simulink model "Planar_Full_System_NL"  (R2016a)
settings: Solver=ode45  StartTime=0.0  StopTime=2  RelTol=1e-3
values from neighbouring files (symbols this model uses):
  T_x_AP = 0    [Computation.m]
  T_y_AP = 0    [Computation.m]
  T_z_AP = 0    [Computation.m]
  x_AP = [0;0;0;0]    [Computation.m]
undefined symbols (not defined in the file or in its folder): K_xz, K_yz
settings Model: Creator=Florian  LastModifiedBy=Florian

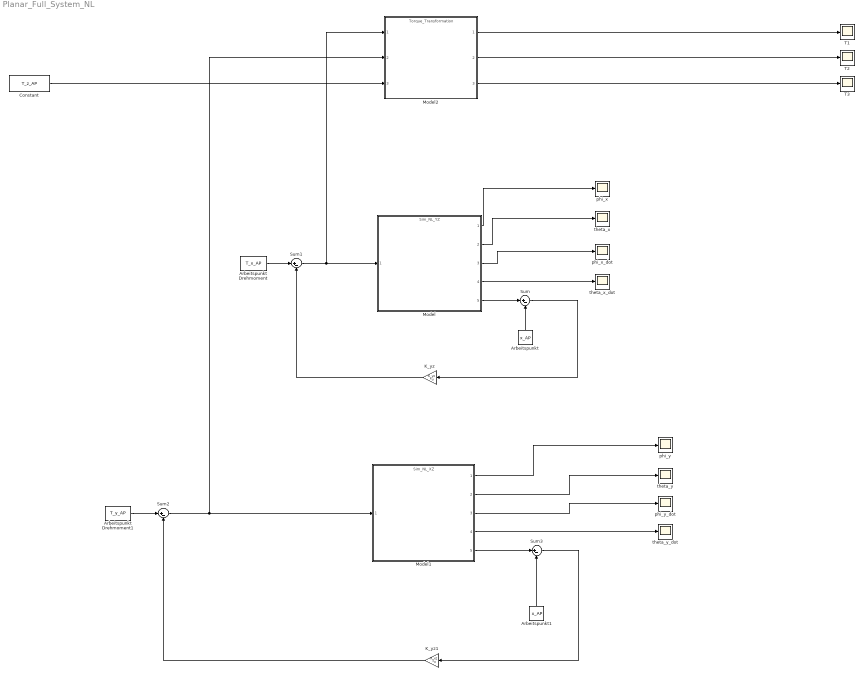
== system Planar_Full_System_NL ==
  Arbeitspunkt : Constant  Value=x_AP
  Arbeitspunkt Drehmoment : Constant  Value=T_x_AP
  Arbeitspunkt Drehmoment1 : Constant  Value=T_y_AP
  Arbeitspunkt1 : Constant  Value=x_AP
  Constant : Constant  Value=T_z_AP
  K_yz : Gain  Gain=K_yz  Multiplication=Matrix(K*u) (u vector)
  K_yz1 : Gain  Gain=K_xz  Multiplication=Matrix(K*u) (u vector)
  Model : ModelReference  ModelNameDialog=Sim_NL_YZ.slx  SimulationMode=Normal  ModelReferenceVersion=1.22
  Model1 : ModelReference  ModelNameDialog=Sim_NL_XZ.slx  SimulationMode=Normal  ModelReferenceVersion=1.4
  Model2 : ModelReference  ModelNameDialog=Torque_Transformation.slx  SimulationMode=Normal  ModelReferenceVersion=1.4
  Sum{,1..3} (4 alike) : Sum  Inputs=|+-
  T1 : Scope
  T2 : Scope
  T3 : Scope
  phi_x : Scope
  phi_x_dot : Scope
  phi_y : Scope
  phi_y_dot : Scope
  theta_x : Scope
  theta_x_dot : Scope
  theta_y : Scope
  theta_y_dot : Scope
  wires:
  Model/1 -> phi_x/1
  Model/2 -> theta_x/1
  Model/3 -> phi_x_dot/1
  Model/4 -> theta_x_dot/1
  Model/5 -> Sum/1
  Sum/1 -> K_yz/1
  Sum1/1 -> Model2/1, Model/1
  K_yz/1 -> Sum1/2
  Arbeitspunkt Drehmoment/1 -> Sum1/1
  Arbeitspunkt/1 -> Sum/2
  Arbeitspunkt Drehmoment1/1 -> Sum2/1
  Sum2/1 -> Model1/1, Model2/2
  Model1/5 -> Sum3/1
  Arbeitspunkt1/1 -> Sum3/2
  Sum3/1 -> K_yz1/1
  K_yz1/1 -> Sum2/2
  Model1/1 -> phi_y/1
  Model1/4 -> theta_y_dot/1
  Model1/3 -> phi_y_dot/1
  Model1/2 -> theta_y/1
  Model2/1 -> T1/1
  Model2/2 -> T2/1
  Model2/3 -> T3/1
  Constant/1 -> Model2/3
